simulink model "simulinkfd123"  (R2015a)
settings: Solver=ode45  StartTime=0.0  StopTime=10.0  RelTol=1e-3
libraries: dsparch4 x1
settings Model: Creator=aluno  LastModifiedBy=aluno

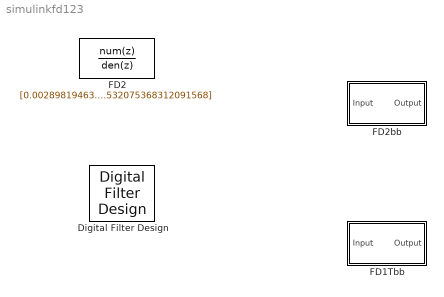
== system simulinkfd123 ==
  Digital Filter Design : dsparch4/Digital Filter Design  mwdsp_browser_bugfix_var=off
  "FD1Tbb " : Subsystem  Tag=FilterWizardSubSystem
      settings: ErrorFcn=dspFilterRealizedInBasicElemsAlgLoopErrFcnCallback
  "FD2 " : DiscreteFilter  Tag=BlockMethodSubSystem  Numerator=[0.00289819463372141843 0 -0.00869458390116425485 0 0.00869458390116425485 0 -0.00289819463372141843]  Denominator=[1 0.851172988233437566 2.61686206988090397 1.38638472726139583 2.12575188112322433 0.558397296097729701 0.532075368312091568]  InputProcessing=Columns as channels (frame based)  a0EqualsOne=on
  "FD2bb " : Subsystem  Tag=FilterWizardSubSystem
      settings: ErrorFcn=dspFilterRealizedInBasicElemsAlgLoopErrFcnCallback

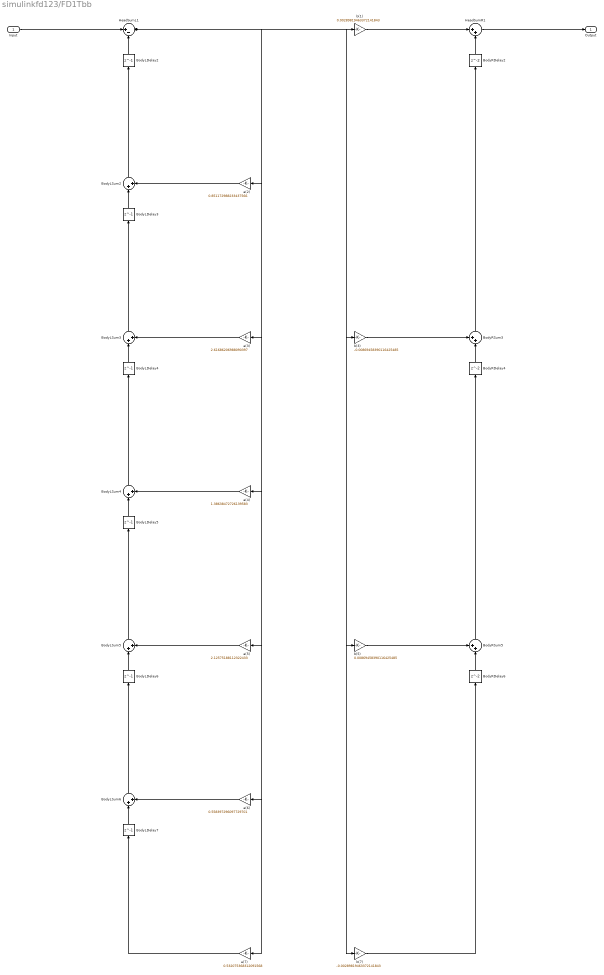
== system simulinkfd123/FD1Tbb  ==
  Input : Inport
  BodyLDelay{2..7} (6 alike) : Delay  DelayLength=1  InitialCondition=0
  BodyLSum{2..6} (5 alike) : Sum  Inputs=|++  RndMeth=Nearest  SaturateOnIntegerOverflow=on  OutDataTypeStr=Inherit: Same as first input
  BodyRDelay2 : Delay  InitialCondition=0
  BodyRDelay4 : Delay  InitialCondition=0
  BodyRDelay6 : Delay  InitialCondition=0
  BodyRSum3 : Sum  Inputs=++|  RndMeth=Nearest  SaturateOnIntegerOverflow=on  OutDataTypeStr=Inherit: Same as first input
  BodyRSum5 : Sum  Inputs=++|  RndMeth=Nearest  SaturateOnIntegerOverflow=on  OutDataTypeStr=Inherit: Same as first input
  HeadSumL1 : Sum  Inputs=|+-  RndMeth=Nearest  SaturateOnIntegerOverflow=on  OutDataTypeStr=Inherit: Same as first input
  HeadSumR1 : Sum  Inputs=|++  RndMeth=Nearest  SaturateOnIntegerOverflow=on  OutDataTypeStr=Inherit: Same as first input
  a(2) : Gain  Gain=0.851172988233437566  ParamDataTypeStr=double  RndMeth=Nearest  SaturateOnIntegerOverflow=on  OutDataTypeStr=Inherit: Same as input
  a(3) : Gain  Gain=2.61686206988090397  ParamDataTypeStr=double  RndMeth=Nearest  SaturateOnIntegerOverflow=on  OutDataTypeStr=Inherit: Same as input
  a(4) : Gain  Gain=1.38638472726139583  ParamDataTypeStr=double  RndMeth=Nearest  SaturateOnIntegerOverflow=on  OutDataTypeStr=Inherit: Same as input
  a(5) : Gain  Gain=2.12575188112322433  ParamDataTypeStr=double  RndMeth=Nearest  SaturateOnIntegerOverflow=on  OutDataTypeStr=Inherit: Same as input
  a(6) : Gain  Gain=0.558397296097729701  ParamDataTypeStr=double  RndMeth=Nearest  SaturateOnIntegerOverflow=on  OutDataTypeStr=Inherit: Same as input
  a(7) : Gain  Gain=0.532075368312091568  ParamDataTypeStr=double  RndMeth=Nearest  SaturateOnIntegerOverflow=on  OutDataTypeStr=Inherit: Same as input
  b(1) : Gain  Gain=0.00289819463372141843  ParamDataTypeStr=double  RndMeth=Nearest  SaturateOnIntegerOverflow=on  OutDataTypeStr=Inherit: Same as input
  b(3) : Gain  Gain=-0.00869458390116425485  ParamDataTypeStr=double  RndMeth=Nearest  SaturateOnIntegerOverflow=on  OutDataTypeStr=Inherit: Same as input
  b(5) : Gain  Gain=0.00869458390116425485  ParamDataTypeStr=double  RndMeth=Nearest  SaturateOnIntegerOverflow=on  OutDataTypeStr=Inherit: Same as input
  b(7) : Gain  Gain=-0.00289819463372141843  ParamDataTypeStr=double  RndMeth=Nearest  SaturateOnIntegerOverflow=on  OutDataTypeStr=Inherit: Same as input
  Output : Outport
  wires:
  Input/1 -> HeadSumL1/1
  HeadSumL1/1 -> b(1)/1, a(2)/1, a(3)/1, a(4)/1, a(5)/1, a(6)/1, a(7)/1, b(3)/1, b(5)/1, b(7)/1
  b(1)/1 -> HeadSumR1/1
  HeadSumR1/1 -> Output/1
  BodyLDelay2/1 -> HeadSumL1/2
  BodyLSum2/1 -> BodyLDelay2/1
  a(2)/1 -> BodyLSum2/2
  BodyRDelay2/1 -> HeadSumR1/2
  BodyLDelay3/1 -> BodyLSum2/1
  BodyLSum3/1 -> BodyLDelay3/1
  a(3)/1 -> BodyLSum3/2
  b(3)/1 -> BodyRSum3/1
  BodyRSum3/1 -> BodyRDelay2/1
  BodyLDelay4/1 -> BodyLSum3/1
  BodyLSum4/1 -> BodyLDelay4/1
  a(4)/1 -> BodyLSum4/2
  BodyRDelay4/1 -> BodyRSum3/2
  BodyLDelay5/1 -> BodyLSum4/1
  BodyLSum5/1 -> BodyLDelay5/1
  a(5)/1 -> BodyLSum5/2
  b(5)/1 -> BodyRSum5/1
  BodyRSum5/1 -> BodyRDelay4/1
  BodyLDelay6/1 -> BodyLSum5/1
  BodyLSum6/1 -> BodyLDelay6/1
  a(6)/1 -> BodyLSum6/2
  BodyRDelay6/1 -> BodyRSum5/2
  BodyLDelay7/1 -> BodyLSum6/1
  a(7)/1 -> BodyLDelay7/1
  b(7)/1 -> BodyRDelay6/1

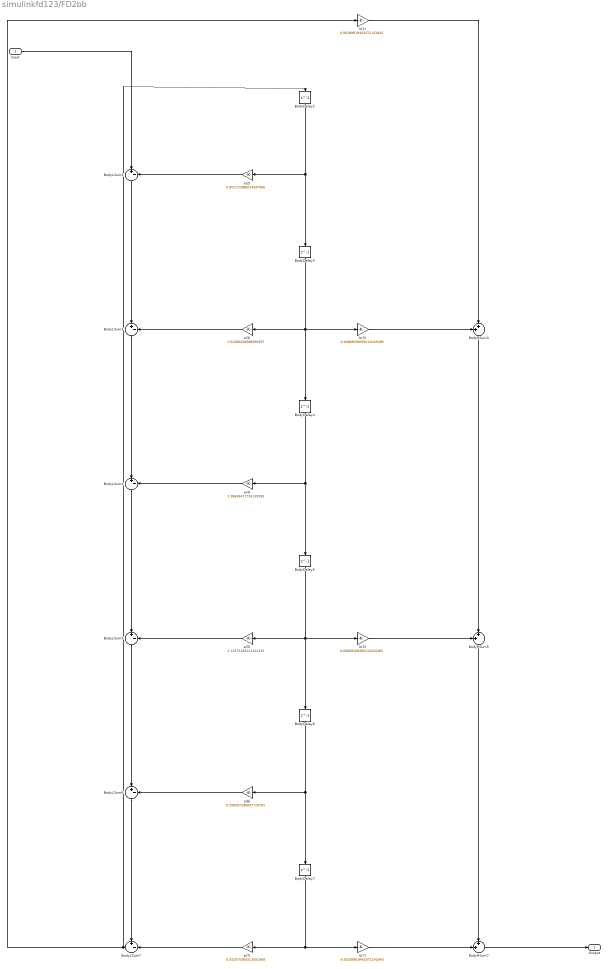
== system simulinkfd123/FD2bb  ==
  Input : Inport
  BodyDelay{2..7} (6 alike) : Delay  DelayLength=1  InitialCondition=0
  BodyLSum{2..6} (5 alike) : Sum  Inputs=|+-  RndMeth=Nearest  SaturateOnIntegerOverflow=on  OutDataTypeStr=Inherit: Same as first input
  BodyLSum7 : Sum  Inputs=+-|  RndMeth=Nearest  SaturateOnIntegerOverflow=on  OutDataTypeStr=Inherit: Same as first input
  BodyRSum3 : Sum  Inputs=++|  RndMeth=Nearest  SaturateOnIntegerOverflow=on  OutDataTypeStr=Inherit: Same as first input
  BodyRSum5 : Sum  Inputs=++|  RndMeth=Nearest  SaturateOnIntegerOverflow=on  OutDataTypeStr=Inherit: Same as first input
  BodyRSum7 : Sum  Inputs=++|  RndMeth=Nearest  SaturateOnIntegerOverflow=on  OutDataTypeStr=Inherit: Same as first input
  a(2) : Gain  Gain=0.851172988233437566  ParamDataTypeStr=double  RndMeth=Nearest  SaturateOnIntegerOverflow=on  OutDataTypeStr=Inherit: Same as input
  a(3) : Gain  Gain=2.61686206988090397  ParamDataTypeStr=double  RndMeth=Nearest  SaturateOnIntegerOverflow=on  OutDataTypeStr=Inherit: Same as input
  a(4) : Gain  Gain=1.38638472726139583  ParamDataTypeStr=double  RndMeth=Nearest  SaturateOnIntegerOverflow=on  OutDataTypeStr=Inherit: Same as input
  a(5) : Gain  Gain=2.12575188112322433  ParamDataTypeStr=double  RndMeth=Nearest  SaturateOnIntegerOverflow=on  OutDataTypeStr=Inherit: Same as input
  a(6) : Gain  Gain=0.558397296097729701  ParamDataTypeStr=double  RndMeth=Nearest  SaturateOnIntegerOverflow=on  OutDataTypeStr=Inherit: Same as input
  a(7) : Gain  Gain=0.532075368312091568  ParamDataTypeStr=double  RndMeth=Nearest  SaturateOnIntegerOverflow=on  OutDataTypeStr=Inherit: Same as input
  b(1) : Gain  Gain=0.00289819463372141843  ParamDataTypeStr=double  RndMeth=Nearest  SaturateOnIntegerOverflow=on  OutDataTypeStr=Inherit: Same as input
  b(3) : Gain  Gain=-0.00869458390116425485  ParamDataTypeStr=double  RndMeth=Nearest  SaturateOnIntegerOverflow=on  OutDataTypeStr=Inherit: Same as input
  b(5) : Gain  Gain=0.00869458390116425485  ParamDataTypeStr=double  RndMeth=Nearest  SaturateOnIntegerOverflow=on  OutDataTypeStr=Inherit: Same as input
  b(7) : Gain  Gain=-0.00289819463372141843  ParamDataTypeStr=double  RndMeth=Nearest  SaturateOnIntegerOverflow=on  OutDataTypeStr=Inherit: Same as input
  Output : Outport
  wires:
  b(1)/1 -> BodyRSum3/2
  Input/1 -> BodyLSum2/1
  BodyLSum2/1 -> BodyLSum3/1
  a(2)/1 -> BodyLSum2/2
  BodyDelay2/1 -> a(2)/1, BodyDelay3/1
  BodyLSum3/1 -> BodyLSum4/1
  a(3)/1 -> BodyLSum3/2
  BodyDelay3/1 -> a(3)/1, b(3)/1, BodyDelay4/1
  b(3)/1 -> BodyRSum3/1
  BodyRSum3/1 -> BodyRSum5/2
  BodyLSum4/1 -> BodyLSum5/1
  a(4)/1 -> BodyLSum4/2
  BodyDelay4/1 -> a(4)/1, BodyDelay5/1
  BodyLSum5/1 -> BodyLSum6/1
  a(5)/1 -> BodyLSum5/2
  BodyDelay5/1 -> a(5)/1, b(5)/1, BodyDelay6/1
  b(5)/1 -> BodyRSum5/1
  BodyRSum5/1 -> BodyRSum7/1
  BodyLSum6/1 -> BodyLSum7/1
  a(6)/1 -> BodyLSum6/2
  BodyDelay6/1 -> a(6)/1, BodyDelay7/1
  BodyLSum7/1 -> b(1)/1, BodyDelay2/1
  a(7)/1 -> BodyLSum7/2
  BodyDelay7/1 -> a(7)/1, b(7)/1
  b(7)/1 -> BodyRSum7/2
  BodyRSum7/1 -> Output/1
